simulink model "Sim6"  (R2021b)
settings: Solver=VariableStepAuto  StartTime=0.0  StopTime=0.1  FixedStep=1e-6  RelTol=1e-6  EnableMultiTasking=on
PreLoadFcn:
  | Ts=5e-6;
InitFcn:
  | Ts=5e-6;
model workspace (MAT data in the model file):
  KipP = 0.53
  KipQ = 0.53
  KppP = 0.1
  KppQ = 0.1
  ki = 1
  kp = 10
  wc = 2
undefined symbols (not defined in the file or in its folder): DiscIntNeverNeededParam
libraries: spsPLL3phLib x1, spsPWMGenerator2LevelLib x1, spsdq0toabcLib x1, spsGroundLib x1, spsThreePhaseProgrammableVoltageSourceLib x1, spsThreePhaseSeriesRLCBranchLib x1, spsThreePhaseVIMeasurementLib x1, spsThreePhaseSourceLib x1, spsUniversalBridgeLib x1, spsDCVoltageSourceLib x1, spspowerguiLib x1
settings Model: SimulationMode=accelerator  Creator=MathWorks  LastModifiedBy=sebastian
settings SolverCC: AlgebraicLoopSolver=TrustRegion  SolverResetMethod=Robust
settings DataIOCC: SaveOutput=off  SignalLogging=off  DSMLogging=off  SaveTime=off  ReturnWorkspaceOutputs=off
settings OptimizationCC: LifeSpan=inf
settings DebuggingCC: ReadBeforeWriteMsg=DisableAll  WriteAfterWriteMsg=DisableAll  WriteAfterReadMsg=DisableAll  MultiTaskDSMMsg=none  SFUnexpectedBacktrackingDiag=warning  SFNoUnconditionalDefaultTransitionDiag=warning  SFExecutionAtInitializationDiag=none  SFMachineParentedDataDiag=warning  ArithmeticOperatorsInVariantConditions=warning
settings ModelReferenceCC: UpdateModelReferenceTargets=IfOutOfDate
settings SFSimCC: SFSimEcho=off  SimUseLocalCustomCode=off  CustomCodeUndefinedFunction=UseInterfaceOnly
settings RTWCC: RTWUseLocalCustomCode=off
settings CodeAppCC: StateflowObjectComments=on
settings GRTTargetCC: TargetLangStandard=C89/C90 (ANSI)
settings ConfigComp: CovMetricSettings=dw  CovSaveCumulativeToWorkspaceVar=on  CovSaveSingleToWorkspaceVar=on  CovExternalEMLEnable=off
settings SimscapeCC: SimscapeNormalizeSystem=off  SimscapeNominalValues={1, 'bar'; 1, 'cm^3/s'; 1, 'bar*kg/s'; 1, 'kJ/kg'; 1, 'kW'; }

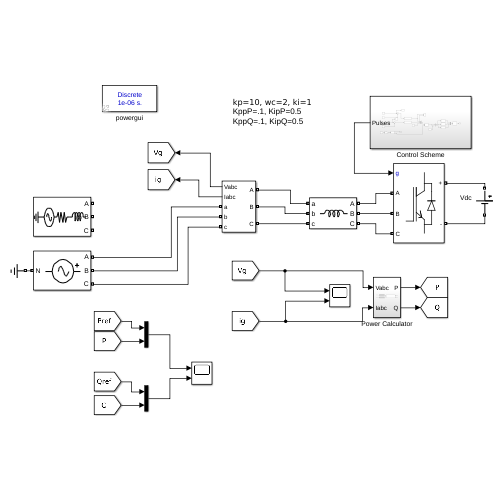
[thumbnail: Simulink's stored preview of the top-level diagram]
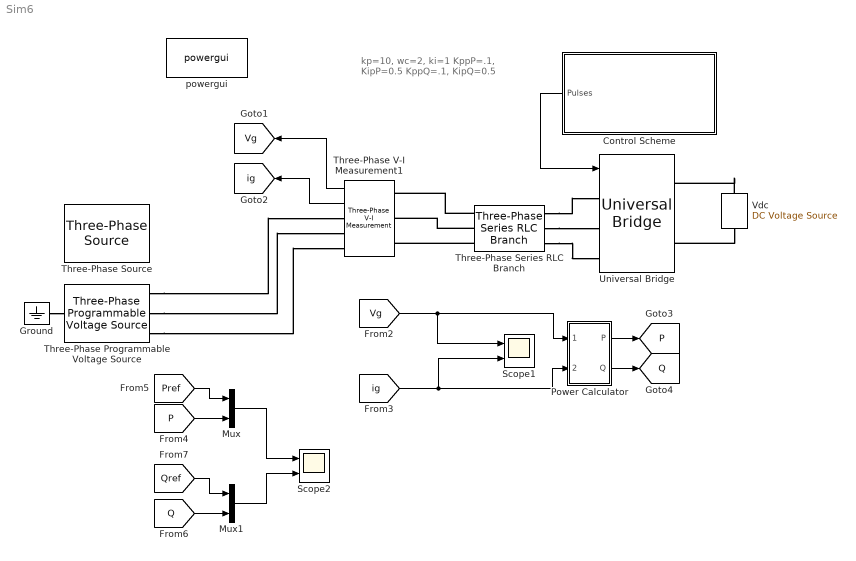
== system Sim6 ==
  note: kp=10, wc=2, ki=1
      | KppP=.1, KipP=0.5
      | KppQ=.1, KipQ=0.5
  Control Scheme : Subsystem
  Ground : spsGroundLib/Ground  LConnTagsString=a
  Mux : Mux  Inputs=2
  Mux1 : Mux  Inputs=2
  Power Calculator : Subsystem
  Scope1 : Scope  NumInputPorts=2
  Scope2 : Scope  NumInputPorts=2
  Three-Phase Programmable Voltage Source : spsThreePhaseProgrammableVoltageSourceLib/Three-Phase Programmable Voltage Source  PositiveSequence="[400  0 50]"  VariationEntity=Amplitude  VariationType=Table of time-amplitude pairs  VariationTypeAlt=Step  VariationStep=0.5  VariationRate=10  VariationMagnitude=0.3  VariationFrequency=2  VariationTiming=[1 2]  VariationPhaseA=off  Amplitudes=[1 0.8 1.2 1.0]  TimeValues=[0 0.1 0.15 0.2]  HarmonicGeneration=on  HarmonicA=[5 0.2 -120 2]  HarmonicB=[7 0.15 0 2]  Timing="[0.05  0.1]"  BusType=swing  Pref=0  Qref=0  Qmin=-inf  Qmax=inf
  Three-Phase Series RLC Branch : spsThreePhaseSeriesRLCBranchLib/Three-Phase Series RLC Branch  LConnTagsString=A|B|C  RConnTagsString=A|B|C  BranchType=L  Resistance=1  Inductance=3e-3  Capacitance=1e-6  Measurements=None
  Three-Phase V-I Measurement1 : spsThreePhaseVIMeasurementLib/Three-Phase V-I Measurement  VoltageMeasurement=phase-to-ground  SetLabelV=off  LabelV=Vabc  Vpu=off  VpuLL=off  CurrentMeasurement=yes  SetLabelI=off  LabelI=Iabc  Ipu=off  Pbase=100e6  Vbase=500e3  OutputType=Complex  PhasorSimulation=off  PSBequivalent=0
  Three-Phase Source : spsThreePhaseSourceLib/Three-Phase Source  InternalConnection=Yg  VoltagePhases=off  Voltage=400  PhaseAngle=0  Voltage_phases=[25e3 25e3 25e3]/sqrt(3)  PhaseAngles_phases=[0 -120 +120]  Frequency=50  NonIdealSource=on  SpecifyImpedance=on  Resistance=0.8929  Inductance=16.58e-3  ShortCircuitLevel=sqrt(3)*400*20000  BaseVoltage=400  XRratio=7  BusType=swing  Pref=10e3  Qref=0  Prefabc=[10e3, 10e3, 10e3]  Qrefabc=[0, 0, 0]  Qmin=-inf  Qmax=inf
  Universal Bridge : spsUniversalBridgeLib/Universal Bridge  Arms=3  SnubberResistance=1e5  SnubberCapacitance=inf  Device=IGBT / Diodes  Ron=1e-3  Lon=0  ForwardVoltages="[  0  0  ]"  ForwardVoltage=0  GTOparameters=[ 10e-6 , 20e-6 ]  IGBTparameters=[ 1e-6 , 2e-6 ]  Measurements=None  Measurements_2=None  converterType=Rectifier
  "Vdc " : spsDCVoltageSourceLib/DC Voltage Source  Amplitude=700  Measurements=None
  powergui : spspowerguiLib/powergui  Priority=1  SimulationMode=Discrete  SampleTime=1e-6  frequency=60  Iterations=50  frequencyindice=50  Pbase=100e6  ErrMax=1e-4  UnitsV=kV  UnitsW=MW  buscounter=0  FunctionMessages=off  echomessages=off  EnableUseOfTLC=off  CurrentSourceSwitches=off  DisableSnubberDevices=off  DisableRonSwitches=off  DisableVfSwitches=off  DisplayEquations=off  AutomaticDiscreteSolvers=off  SolverType=Tustin/Backward Euler (TBE)  Interpol=off  ExternalGateDelay=off  methode=off  Ts=100  x0status=blocks  SPID=off  SwTol=0  HookPort=off  NonlinearTolerance=1e-4  nMaxIteration=100  ContinueOnMaxIteration=off  RestoreLinks=warning  ResistiveCurrentMeasurement=off  Frange=[0:2:500]  Ylog=off  Xlog=on  ShowGrid=off  save=off  variable=ZData  structure=ScopeData2  ZoomFFT=off  StartTime=.07-1/50  cycles=1  DisplayStyle=1  fundamental=50  FreqAxis=off  MaxFrequency=1300  frequencyindicesteady=1  RmsSteady=1  display=off
  tag scope: P=global, Q=global, Vg=global, ig=global
  wires:
  Control Scheme/1(Pulses) -> Universal Bridge/1
  Three-Phase V-I Measurement1/2 -> [ig]
  Three-Phase V-I Measurement1/1 -> [Vg]
  [ig] -> Scope1/2, Power Calculator/2(Iabc)
  [Vg] -> Scope1/1, Power Calculator/1(Vabc)
  [P] -> Mux/2
  [Pref] -> Mux/1
  Mux/1 -> Scope2/1
  [Qref] -> Mux1/1
  [Q] -> Mux1/2
  Mux1/1 -> Scope2/2
  Power Calculator/1(P) -> [P]
  Power Calculator/2(Q) -> [Q]
  connections:
  "Vdc "/LConn1 -- Universal Bridge/RConn2
  Three-Phase Series RLC Branch/LConn2 -- Universal Bridge/LConn2
  Three-Phase Series RLC Branch/LConn1 -- Universal Bridge/LConn1
  Three-Phase Series RLC Branch/LConn3 -- Universal Bridge/LConn3
  Three-Phase Series RLC Branch/RConn1 -- Three-Phase V-I Measurement1/LConn1
  Three-Phase Series RLC Branch/RConn2 -- Three-Phase V-I Measurement1/LConn2
  Three-Phase Series RLC Branch/RConn3 -- Three-Phase V-I Measurement1/LConn3
  "Vdc "/RConn1 -- Universal Bridge/RConn1
  Three-Phase Programmable Voltage Source/RConn1 -- Three-Phase V-I Measurement1/RConn1
  Three-Phase Programmable Voltage Source/RConn2 -- Three-Phase V-I Measurement1/RConn2
  Three-Phase Programmable Voltage Source/RConn3 -- Three-Phase V-I Measurement1/RConn3
  Ground/LConn1 -- Three-Phase Programmable Voltage Source/LConn1

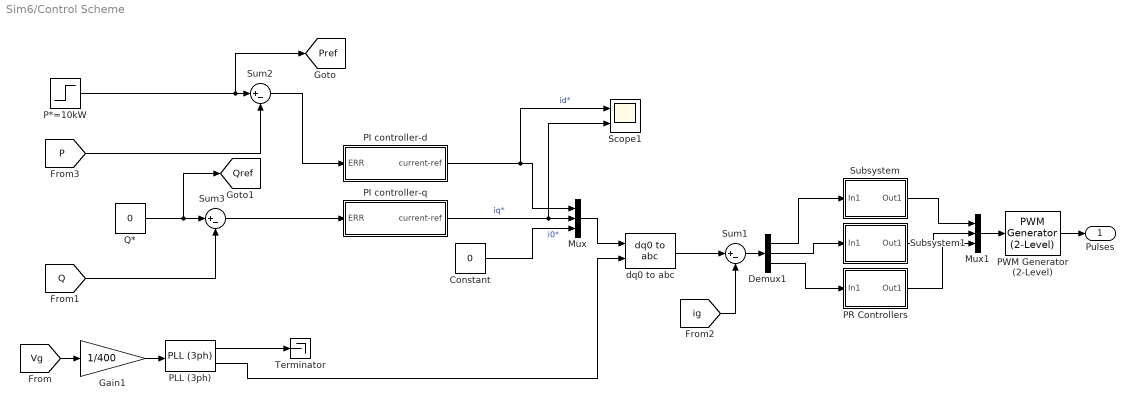
== system Sim6/Control Scheme ==
  Constant : Constant  Value=0
  Demux1 : Demux  Outputs=3
  Gain1 : Gain  Gain=1/400
  Mux : Mux  Inputs=3
  Mux1 : Mux  Inputs=3
  P*=10kW : Step  Time=.05  After=10000  SampleTime=0
  PI controller-d : Subsystem
  PI controller-q : Subsystem
  PLL (3ph) : spsPLL3phLib/PLL (3ph)  Fmin=45  Par_Init=[0, 50]  ParK=[180, 3200, 1]  TcD=1e-4  MaxRateChangeFreq=12  FilterCutOffFreq=25  Ts=0  AGC=on
  PR Controllers : Subsystem
  PWM Generator (2-Level) : spsPWMGenerator2LevelLib/PWM Generator (2-Level)  ModulatorType=Three-phase bridge (6 pulses)  ModulatorMode=Unsynchronized  Fc=20000  Pc=90  nF=27  MinMax="[ -1  1 ]"  SamplingTechnique=Natural  ModulatingSignals=off  m=0.8  Freq=60  Phase=0  Ts=0  ShowCarrierOutport=off
  Q* : Constant  Value=0
  Scope1 : Scope  NumInputPorts=2
  Subsystem : Subsystem
  Subsystem1 : Subsystem
  Sum1 : Sum  Inputs=|+-
  Sum2 : Sum  Inputs=|+-
  Sum3 : Sum  Inputs=|+-
  Terminator : Terminator
  dq0 to abc : spsdq0toabcLib/dq0 to abc  Alignment=90 degrees behind phase A axis
  Pulses : Outport
  tag scope: Pref=global, Qref=global
  wires:
  [Vg] -> Gain1/1
  Gain1/1 -> PLL (3ph)/1
  Constant/1 -> Mux/3  "i0*"
  Mux/1 -> dq0 to abc/1
  dq0 to abc/1 -> Sum1/1
  [ig] -> Sum1/2
  Sum1/1 -> Demux1/1
  PWM Generator (2-Level)/1 -> Pulses/1
  Demux1/1 -> Subsystem/1(In1)
  Demux1/3 -> PR Controllers/1(In1)
  Demux1/2 -> Subsystem1/1(In1)
  Mux1/1 -> PWM Generator (2-Level)/1
  Subsystem/1(Out1) -> Mux1/1
  Subsystem1/1(Out1) -> Mux1/2
  PR Controllers/1(Out1) -> Mux1/3
  PLL (3ph)/1 -> Terminator/1
  PLL (3ph)/2 -> dq0 to abc/2
  PI controller-q/1(current-ref) -> Scope1/2, Mux/2  "iq*"
  PI controller-d/1(current-ref) -> Scope1/1, Mux/1  "id*"
  Q*/1 -> [Qref], Sum3/1
  [Q] -> Sum3/2
  [P] -> Sum2/2
  Sum2/1 -> PI controller-d/1(ERR)
  Sum3/1 -> PI controller-q/1(ERR)
  P*=10kW/1 -> [Pref], Sum2/1

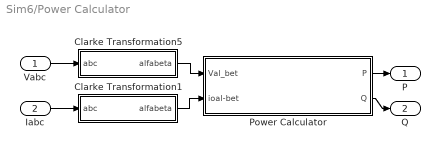
== system Sim6/Power Calculator ==
  Vabc : Inport
  Iabc : Inport  Port=2
  Clarke Transformation1 : Subsystem
  Clarke Transformation5 : Subsystem
  Power Calculator : Subsystem
  P : Outport
  Q : Outport  Port=2
  wires:
  Power Calculator/1(P) -> P/1
  Clarke Transformation1/1(alfabeta) -> Power Calculator/2(ioal-bet)
  Vabc/1 -> Clarke Transformation5/1(abc)
  Clarke Transformation5/1(alfabeta) -> Power Calculator/1(Val_bet)
  Power Calculator/2(Q) -> Q/1
  Iabc/1 -> Clarke Transformation1/1(abc)

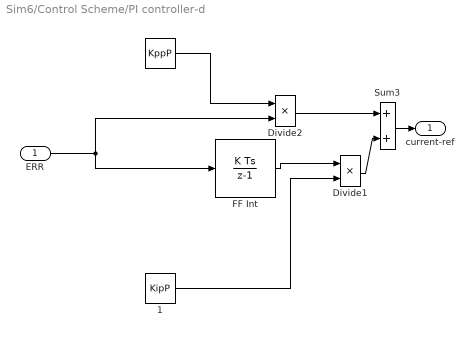
== system Sim6/Control Scheme/PI controller-d ==
  ERR : Inport
  " " : Constant  Value=KppP
  " 1" : Constant  Value=KipP
  Divide1 : Product  Inputs=**  SampleTime=Ts  OutDataTypeStr=Inherit: Same as first input
  Divide2 : Product  Inputs=**  SampleTime=Ts  OutDataTypeStr=Inherit: Same as first input
  FF Int : DiscreteIntegrator  SampleTime=-1  ICPrevOutput=DiscIntNeverNeededParam  ICPrevScaledInput=DiscIntNeverNeededParam
  Sum3 : Sum  OutDataTypeStr=Inherit: Same as first input
  current-ref : Outport
  wires:
  Sum3/1 -> current-ref/1
  Divide1/1 -> Sum3/2
  Divide2/1 -> Sum3/1
  FF Int/1 -> Divide1/1
  ERR/1 -> FF Int/1, Divide2/2
  " "/1 -> Divide2/1
  " 1"/1 -> Divide1/2

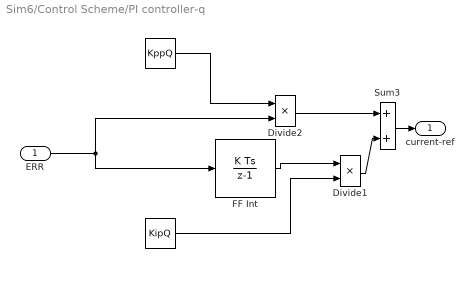
== system Sim6/Control Scheme/PI controller-q ==
  ERR : Inport
  " " : Constant  Value=KppQ
  "   " : Constant  Value=KipQ
  Divide1 : Product  Inputs=**  SampleTime=Ts  OutDataTypeStr=Inherit: Same as first input
  Divide2 : Product  Inputs=**  SampleTime=Ts  OutDataTypeStr=Inherit: Same as first input
  FF Int : DiscreteIntegrator  SampleTime=-1  ICPrevOutput=DiscIntNeverNeededParam  ICPrevScaledInput=DiscIntNeverNeededParam
  Sum3 : Sum  OutDataTypeStr=Inherit: Same as first input
  current-ref : Outport
  wires:
  "   "/1 -> Divide1/2
  " "/1 -> Divide2/1
  ERR/1 -> Divide2/2, FF Int/1
  FF Int/1 -> Divide1/1
  Divide2/1 -> Sum3/1
  Divide1/1 -> Sum3/2
  Sum3/1 -> current-ref/1

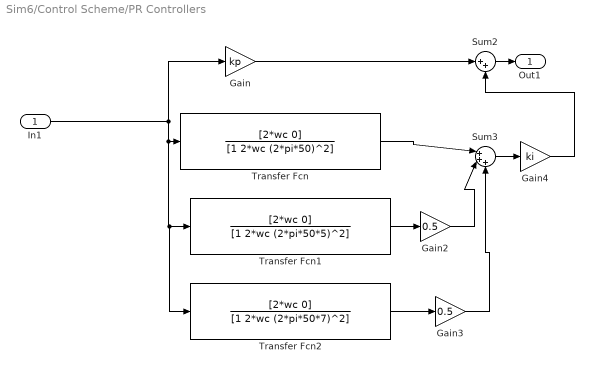
== system Sim6/Control Scheme/PR Controllers ==
  In1 : Inport
  Gain : Gain  Gain=kp
  Gain2 : Gain  Gain=0.5
  Gain3 : Gain  Gain=0.5
  Gain4 : Gain  Gain=ki
  Sum2 : Sum  Inputs=|++
  Sum3 : Sum  Inputs=|+++
  Transfer Fcn : TransferFcn  Numerator=[2*wc 0]  Denominator=[1 2*wc (2*pi*50)^2]
  Transfer Fcn1 : TransferFcn  Numerator=[2*wc 0]  Denominator=[1 2*wc (2*pi*50*5)^2]
  Transfer Fcn2 : TransferFcn  Numerator=[2*wc 0]  Denominator=[1 2*wc (2*pi*50*7)^2]
  Out1 : Outport
  wires:
  Transfer Fcn/1 -> Sum3/1
  Gain/1 -> Sum2/1
  In1/1 -> Transfer Fcn2/1, Transfer Fcn1/1, Transfer Fcn/1, Gain/1
  Gain2/1 -> Sum3/2
  Gain4/1 -> Sum2/2
  Gain3/1 -> Sum3/3
  Transfer Fcn2/1 -> Gain3/1
  Sum3/1 -> Gain4/1
  Transfer Fcn1/1 -> Gain2/1
  Sum2/1 -> Out1/1

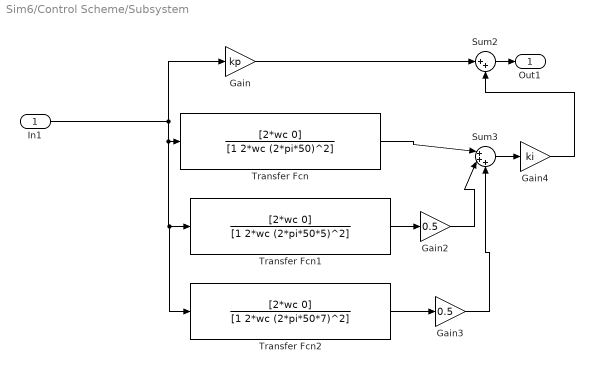
== system Sim6/Control Scheme/Subsystem ==
  In1 : Inport
  Gain : Gain  Gain=kp
  Gain2 : Gain  Gain=0.5
  Gain3 : Gain  Gain=0.5
  Gain4 : Gain  Gain=ki
  Sum2 : Sum  Inputs=|++
  Sum3 : Sum  Inputs=|+++
  Transfer Fcn : TransferFcn  Numerator=[2*wc 0]  Denominator=[1 2*wc (2*pi*50)^2]
  Transfer Fcn1 : TransferFcn  Numerator=[2*wc 0]  Denominator=[1 2*wc (2*pi*50*5)^2]
  Transfer Fcn2 : TransferFcn  Numerator=[2*wc 0]  Denominator=[1 2*wc (2*pi*50*7)^2]
  Out1 : Outport
  wires:
  Transfer Fcn/1 -> Sum3/1
  Gain/1 -> Sum2/1
  In1/1 -> Transfer Fcn2/1, Transfer Fcn1/1, Transfer Fcn/1, Gain/1
  Gain2/1 -> Sum3/2
  Gain4/1 -> Sum2/2
  Gain3/1 -> Sum3/3
  Transfer Fcn2/1 -> Gain3/1
  Sum3/1 -> Gain4/1
  Transfer Fcn1/1 -> Gain2/1
  Sum2/1 -> Out1/1

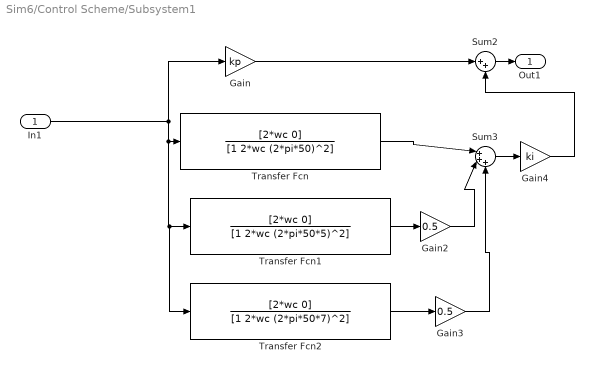
== system Sim6/Control Scheme/Subsystem1 ==
  In1 : Inport
  Gain : Gain  Gain=kp
  Gain2 : Gain  Gain=0.5
  Gain3 : Gain  Gain=0.5
  Gain4 : Gain  Gain=ki
  Sum2 : Sum  Inputs=|++
  Sum3 : Sum  Inputs=|+++
  Transfer Fcn : TransferFcn  Numerator=[2*wc 0]  Denominator=[1 2*wc (2*pi*50)^2]
  Transfer Fcn1 : TransferFcn  Numerator=[2*wc 0]  Denominator=[1 2*wc (2*pi*50*5)^2]
  Transfer Fcn2 : TransferFcn  Numerator=[2*wc 0]  Denominator=[1 2*wc (2*pi*50*7)^2]
  Out1 : Outport
  wires:
  Transfer Fcn/1 -> Sum3/1
  Gain/1 -> Sum2/1
  In1/1 -> Transfer Fcn2/1, Transfer Fcn1/1, Transfer Fcn/1, Gain/1
  Gain2/1 -> Sum3/2
  Gain4/1 -> Sum2/2
  Gain3/1 -> Sum3/3
  Transfer Fcn2/1 -> Gain3/1
  Sum3/1 -> Gain4/1
  Transfer Fcn1/1 -> Gain2/1
  Sum2/1 -> Out1/1

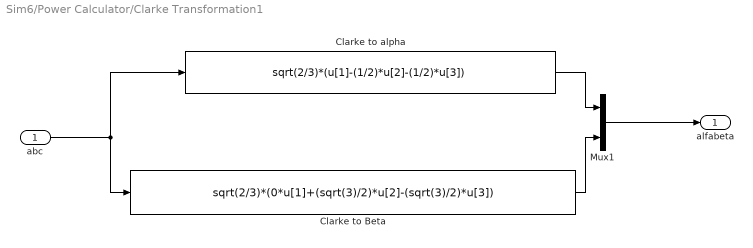
== system Sim6/Power Calculator/Clarke Transformation1 ==
  abc : Inport  SampleTime=Ts
  Clarke to Beta : Fcn  Expr=sqrt(2/3)*(0*u[1]+(sqrt(3)/2)*u[2]-(sqrt(3)/2)*u[3])  SampleTime=Ts
  Clarke to alpha : Fcn  Expr=sqrt(2/3)*(u[1]-(1/2)*u[2]-(1/2)*u[3])  SampleTime=Ts
  Mux1 : Mux  Inputs=2
  alfabeta : Outport  SampleTime=Ts
  wires:
  Clarke to Beta/1 -> Mux1/2
  Clarke to alpha/1 -> Mux1/1
  Mux1/1 -> alfabeta/1
  abc/1 -> Clarke to alpha/1, Clarke to Beta/1

== system Sim6/Power Calculator/Clarke Transformation5 ==
  abc : Inport
  Clarke to Beta : Fcn  Expr=sqrt(2/3)*(0*u[1]+(sqrt(3)/2)*u[2]-(sqrt(3)/2)*u[3])
  Clarke to alpha : Fcn  Expr=sqrt(2/3)*(u[1]-(1/2)*u[2]-(1/2)*u[3])
  Mux1 : Mux  Inputs=2
  alfabeta : Outport
  wires:
  abc/1 -> Clarke to Beta/1, Clarke to alpha/1
  Mux1/1 -> alfabeta/1
  Clarke to alpha/1 -> Mux1/1
  Clarke to Beta/1 -> Mux1/2

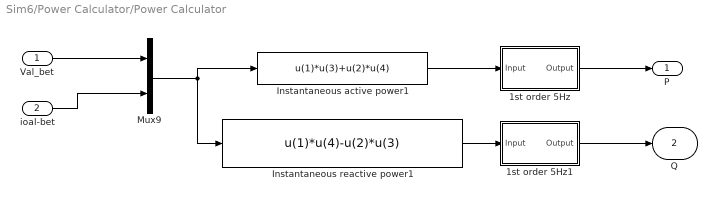
== system Sim6/Power Calculator/Power Calculator ==
  Val_bet : Inport
  ioal-bet : Inport  Port=2
  1st order 5Hz : Subsystem  Tag=FilterWizardSubSystem
      settings: ErrorFcn=dspFilterRealizedInBasicElemsAlgLoopErrFcnCallback
  1st order 5Hz1 : Subsystem  Tag=FilterWizardSubSystem
      settings: ErrorFcn=dspFilterRealizedInBasicElemsAlgLoopErrFcnCallback
  Instantaneous active power1 : Fcn  Expr=u(1)*u(3)+u(2)*u(4)
  Instantaneous reactive power1 : Fcn  Expr=u(1)*u(4)-u(2)*u(3)
  Mux9 : Mux  Inputs=2
  P : Outport
  Q : Outport  Port=2
  wires:
  Mux9/1 -> Instantaneous active power1/1, Instantaneous reactive power1/1
  Val_bet/1 -> Mux9/1
  ioal-bet/1 -> Mux9/2
  Instantaneous active power1/1 -> 1st order 5Hz/1(Input)
  1st order 5Hz/1(Output) -> P/1
  Instantaneous reactive power1/1 -> 1st order 5Hz1/1(Input)
  1st order 5Hz1/1(Output) -> Q/1

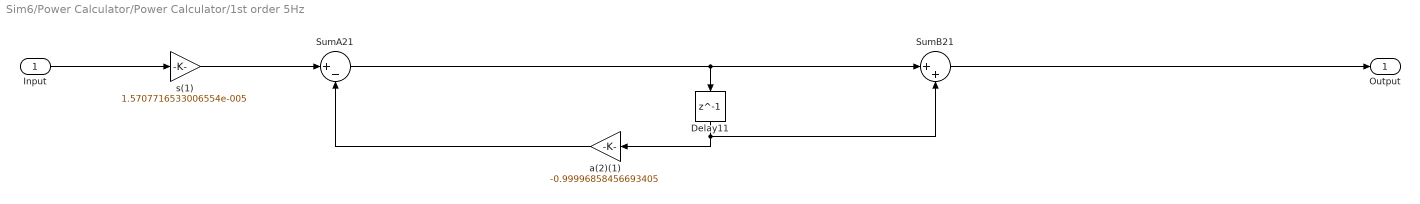
== system Sim6/Power Calculator/Power Calculator/1st order 5Hz ==
  Input : Inport
  Delay11 : Delay  DelayLength=1  InitialCondition=0
  SumA21 : Sum  Inputs=|+-  RndMeth=Nearest  SaturateOnIntegerOverflow=on  OutDataTypeStr=Inherit: Same as first input
  SumB21 : Sum  Inputs=|++  RndMeth=Nearest  SaturateOnIntegerOverflow=on  OutDataTypeStr=Inherit: Same as first input
  a(2)(1) : Gain  Gain=-0.99996858456693405  ParamDataTypeStr=float('double')  RndMeth=Nearest  SaturateOnIntegerOverflow=on  OutDataTypeStr=Inherit: Same as input
  s(1) : Gain  Gain=1.5707716533006554e-005  ParamDataTypeStr=float('double')  RndMeth=Nearest  SaturateOnIntegerOverflow=on  OutDataTypeStr=Inherit: Same as input
  Output : Outport
  wires:
  Input/1 -> s(1)/1
  s(1)/1 -> SumA21/1
  SumA21/1 -> SumB21/1, Delay11/1
  SumB21/1 -> Output/1
  a(2)(1)/1 -> SumA21/2
  Delay11/1 -> a(2)(1)/1, SumB21/2

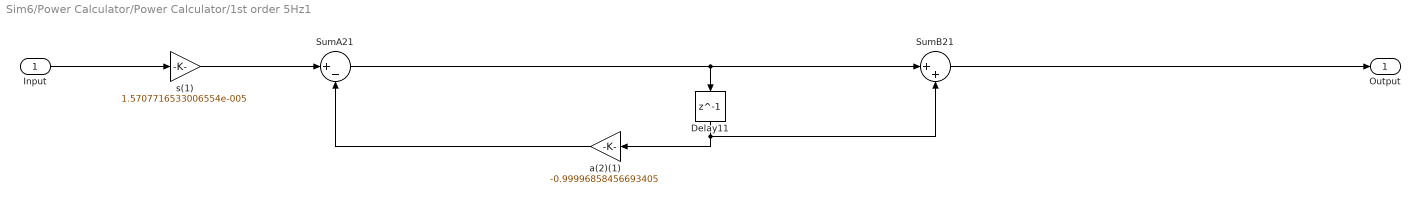
== system Sim6/Power Calculator/Power Calculator/1st order 5Hz1 ==
  Input : Inport
  Delay11 : Delay  DelayLength=1  InitialCondition=0
  SumA21 : Sum  Inputs=|+-  RndMeth=Nearest  SaturateOnIntegerOverflow=on  OutDataTypeStr=Inherit: Same as first input
  SumB21 : Sum  Inputs=|++  RndMeth=Nearest  SaturateOnIntegerOverflow=on  OutDataTypeStr=Inherit: Same as first input
  a(2)(1) : Gain  Gain=-0.99996858456693405  ParamDataTypeStr=float('double')  RndMeth=Nearest  SaturateOnIntegerOverflow=on  OutDataTypeStr=Inherit: Same as input
  s(1) : Gain  Gain=1.5707716533006554e-005  ParamDataTypeStr=float('double')  RndMeth=Nearest  SaturateOnIntegerOverflow=on  OutDataTypeStr=Inherit: Same as input
  Output : Outport
  wires:
  Delay11/1 -> SumB21/2, a(2)(1)/1
  a(2)(1)/1 -> SumA21/2
  SumB21/1 -> Output/1
  SumA21/1 -> Delay11/1, SumB21/1
  s(1)/1 -> SumA21/1
  Input/1 -> s(1)/1
